simulink model "generic_20231123_1032"  (R2022b)
settings: Solver=ode45  StartTime=0.0  StopTime=50  RelTol=1e-3  EnableMultiTasking=on
model workspace (MAT data in the model file):
  A = 1
  Amplifier = -9.10007585438
  B = 1.19071237887
  K_d_yawrate = 0.231634180251
  K_dsteering = 5.24463953925
  k_speed = -0.570636497542
  k_stanley = 28.4909595466
  kd = -9.99955278144
  ki = 0.00519416981022
  kp = 9.99999979837
  path_curvature = 0
values from neighbouring files (symbols this model uses):
  brake_select = ones(length(speed), length(steering_angle))    [TwoDLook_uptable.m]
  curvature = 0.000:0.001:1    [TwoDLook_uptable.m]
  m = 1600    [MPCController1.m]    (also in MPCController2.m; MPC_Fmincon.m)
  speed = 0:0.1:100    [TwoDLook_uptable.m]
  steering_angle = -3.14/4:0.00628/4:3.14/4    [TwoDLook_uptable.m]
undefined symbols (not defined in the file or in its folder): DiscIntNeverNeededParam
libraries: CarMaker4SL x143, simulink x11, cstblocks x6, simulink_extras x4, autolibshared x1, mpcadaslib x1
(part 5 of 7)

== system generic_20231123_1032/CarMaker/VehicleControl/CreateBus VhclCtrl/Stanley steering & speed//Brake controller/Road sensor set & path planning/Road sensor set & path planning/Dijkestra path planning/Signal_smoothing/Smoothing4 ==
  Signal_In : Inport
  Add : Sum  Inputs=++++
  Delay : Delay  InitialCondition=0.1
  Delay1 : Delay  DelayLength=4  InitialCondition=0.1
  Delay2 : Delay  DelayLength=5  InitialCondition=0.1
  Gain : Gain  Gain=0.35
  Gain1 : Gain  Gain=0.25
  Gain2 : Gain  Gain=0.25
  Gain3 : Gain  Gain=0.15
  Signal_Out : Outport  VectorParamsAs1DForOutWhenUnconnected=off
  wires:
  Gain3/1 -> Add/4
  Delay2/1 -> Gain3/1
  Gain2/1 -> Add/3
  Add/1 -> Signal_Out/1, Delay/1, Delay1/1, Delay2/1
  Delay1/1 -> Gain2/1
  Gain/1 -> Add/1
  Delay/1 -> Gain1/1
  Signal_In/1 -> Gain/1
  Gain1/1 -> Add/2

== system generic_20231123_1032/CarMaker/VehicleControl/CreateBus VhclCtrl/Stanley steering & speed//Brake controller/Road sensor set & path planning/Road sensor set & path planning/Spline_path_planning/Signal_smoothing/Smoothing1 ==
  Signal_In : Inport
  Add : Sum  Inputs=++++
  Delay : Delay  InitialCondition=0.1
  Delay1 : Delay  DelayLength=4  InitialCondition=0.1
  Delay2 : Delay  DelayLength=5  InitialCondition=0.1
  Gain : Gain  Gain=0.35
  Gain1 : Gain  Gain=0.25
  Gain2 : Gain  Gain=0.25
  Gain3 : Gain  Gain=0.15
  Signal_Out : Outport  VectorParamsAs1DForOutWhenUnconnected=off
  wires:
  Gain1/1 -> Add/2
  Signal_In/1 -> Gain/1
  Delay/1 -> Gain1/1
  Gain/1 -> Add/1
  Delay1/1 -> Gain2/1
  Add/1 -> Delay2/1, Delay1/1, Delay/1, Signal_Out/1
  Gain2/1 -> Add/3
  Delay2/1 -> Gain3/1
  Gain3/1 -> Add/4

== system generic_20231123_1032/CarMaker/VehicleControl/CreateBus VhclCtrl/Stanley steering & speed//Brake controller/Road sensor set & path planning/Road sensor set & path planning/Spline_path_planning/Signal_smoothing/Smoothing2 ==
  Signal_In : Inport
  Add : Sum  Inputs=++++
  Delay : Delay  InitialCondition=0.1
  Delay1 : Delay  DelayLength=4  InitialCondition=0.1
  Delay2 : Delay  DelayLength=5  InitialCondition=0.1
  Gain : Gain  Gain=0.35
  Gain1 : Gain  Gain=0.25
  Gain2 : Gain  Gain=0.25
  Gain3 : Gain  Gain=0.15
  Signal_Out : Outport  VectorParamsAs1DForOutWhenUnconnected=off
  wires:
  Gain3/1 -> Add/4
  Delay2/1 -> Gain3/1
  Gain2/1 -> Add/3
  Add/1 -> Signal_Out/1, Delay/1, Delay1/1, Delay2/1
  Delay1/1 -> Gain2/1
  Gain/1 -> Add/1
  Delay/1 -> Gain1/1
  Signal_In/1 -> Gain/1
  Gain1/1 -> Add/2

== system generic_20231123_1032/CarMaker/VehicleControl/CreateBus VhclCtrl/Stanley steering & speed//Brake controller/Road sensor set & path planning/Road sensor set & path planning/Spline_path_planning/Signal_smoothing/Smoothing4 ==
  Signal_In : Inport
  Add : Sum  Inputs=++++
  Delay : Delay  InitialCondition=0.1
  Delay1 : Delay  DelayLength=4  InitialCondition=0.1
  Delay2 : Delay  DelayLength=5  InitialCondition=0.1
  Gain : Gain  Gain=0.35
  Gain1 : Gain  Gain=0.25
  Gain2 : Gain  Gain=0.25
  Gain3 : Gain  Gain=0.15
  Signal_Out : Outport  VectorParamsAs1DForOutWhenUnconnected=off
  wires:
  Gain1/1 -> Add/2
  Signal_In/1 -> Gain/1
  Delay/1 -> Gain1/1
  Gain/1 -> Add/1
  Delay1/1 -> Gain2/1
  Add/1 -> Delay2/1, Delay1/1, Delay/1, Signal_Out/1
  Gain2/1 -> Add/3
  Delay2/1 -> Gain3/1
  Gain3/1 -> Add/4

== system generic_20231123_1032/CarMaker/VehicleControl/CreateBus VhclCtrl/Stanley steering & speed//Brake controller/Road sensor set & path planning/Road sensor set & path planning/path_planning/Signal_smoothing/Smoothing1 ==
  Signal_In : Inport
  Add : Sum  Inputs=++++
  Delay : Delay  InitialCondition=0.1
  Delay1 : Delay  DelayLength=4  InitialCondition=0.1
  Delay2 : Delay  DelayLength=5  InitialCondition=0.1
  Gain : Gain  Gain=0.35
  Gain1 : Gain  Gain=0.25
  Gain2 : Gain  Gain=0.25
  Gain3 : Gain  Gain=0.15
  Signal_Out : Outport  VectorParamsAs1DForOutWhenUnconnected=off
  wires:
  Gain3/1 -> Add/4
  Delay2/1 -> Gain3/1
  Gain2/1 -> Add/3
  Add/1 -> Signal_Out/1, Delay/1, Delay1/1, Delay2/1
  Delay1/1 -> Gain2/1
  Gain/1 -> Add/1
  Delay/1 -> Gain1/1
  Signal_In/1 -> Gain/1
  Gain1/1 -> Add/2

== system generic_20231123_1032/CarMaker/VehicleControl/CreateBus VhclCtrl/Stanley steering & speed//Brake controller/Road sensor set & path planning/Road sensor set & path planning/path_planning/Signal_smoothing/Smoothing2 ==
  Signal_In : Inport
  Add : Sum  Inputs=++++
  Delay : Delay  InitialCondition=0.1
  Delay1 : Delay  DelayLength=4  InitialCondition=0.1
  Delay2 : Delay  DelayLength=5  InitialCondition=0.1
  Gain : Gain  Gain=0.35
  Gain1 : Gain  Gain=0.25
  Gain2 : Gain  Gain=0.25
  Gain3 : Gain  Gain=0.15
  Signal_Out : Outport  VectorParamsAs1DForOutWhenUnconnected=off
  wires:
  Gain1/1 -> Add/2
  Signal_In/1 -> Gain/1
  Delay/1 -> Gain1/1
  Gain/1 -> Add/1
  Delay1/1 -> Gain2/1
  Add/1 -> Delay2/1, Delay1/1, Delay/1, Signal_Out/1
  Gain2/1 -> Add/3
  Delay2/1 -> Gain3/1
  Gain3/1 -> Add/4

== system generic_20231123_1032/CarMaker/VehicleControl/CreateBus VhclCtrl/Stanley steering & speed//Brake controller/Road sensor set & path planning/Road sensor set & path planning/path_planning/Signal_smoothing/Smoothing4 ==
  Signal_In : Inport
  Add : Sum  Inputs=++++
  Delay : Delay  InitialCondition=0.1
  Delay1 : Delay  DelayLength=4  InitialCondition=0.1
  Delay2 : Delay  DelayLength=5  InitialCondition=0.1
  Gain : Gain  Gain=0.35
  Gain1 : Gain  Gain=0.25
  Gain2 : Gain  Gain=0.25
  Gain3 : Gain  Gain=0.15
  Signal_Out : Outport  VectorParamsAs1DForOutWhenUnconnected=off
  wires:
  Gain3/1 -> Add/4
  Delay2/1 -> Gain3/1
  Gain2/1 -> Add/3
  Add/1 -> Signal_Out/1, Delay/1, Delay1/1, Delay2/1
  Delay1/1 -> Gain2/1
  Gain/1 -> Add/1
  Delay/1 -> Gain1/1
  Signal_In/1 -> Gain/1
  Gain1/1 -> Add/2

== system generic_20231123_1032/CarMaker/VehicleControl/CreateBus VhclCtrl/Stanley steering & speed//Brake controller/Stanley_controller_vfin/Stanley_controller_vfin/Stanley_standfort controller/Steady_state_yaw/Steady_state_yaw ==
  V : Inport
  Curvature : Inport  Port=2
  Constant : Constant  Value=1600.004
  Constant1 : Constant  Value=70551.0
  Constant3 : Constant  Value=1.488
  Constant4 : Constant  Value=1.487
  Constant5 : Constant
  Divide : Product  Inputs=*/
  Divide1 : Product  Inputs=*/
  Gain : Gain  Gain=180/pi()
  Product : Product  Inputs=3
  Product1 : Product
  Square : Math  Operator=square
  Sum : Sum  Inputs=|++
  Steady_state_yaw : Outport
  wires:
  Square/1 -> Product/1
  Constant4/1 -> Divide/1
  Constant5/1 -> Sum/1
  Constant3/1 -> Divide/2
  V/1 -> Square/1
  Divide/1 -> Sum/2
  Sum/1 -> Product1/2
  Constant/1 -> Product/2
  Curvature/1 -> Product/3
  Constant1/1 -> Gain/1
  Product/1 -> Divide1/1
  Product1/1 -> Divide1/2
  Divide1/1 -> Steady_state_yaw/1
  Gain/1 -> Product1/1

== matlab function generic_20231123_1032/CarMaker/VehicleControl/Subsystem/MATLAB Function ==
  data: currentPosition input; currentHeading output; nextWaypoint input; desiredHeading output; headingError output
function [currentHeading, desiredHeading, headingError] = calculateHeadingError(currentPosition, nextWaypoint)
    % Calculate current heading, desired heading, and heading error for Stanley controller
    % Inputs:
    %   - currentPosition: Current position of the vehicle [x, y] (single points)
    %   - nextWaypoint: Next waypoint on the path [x, y]
    % Outputs:
    %   - currentHeading: Current heading of the vehicle (in radians)
    %   - desiredHeading: Desired heading or reference angle (in radians)
    %   - headingError: Heading error (in radians)
    function angle = wrapToPi(angle)
    % Wrap angle to the range [-pi, pi]
    angle = mod(angle + pi, 2 * pi) - pi;
    end
    % Extract x and y coordinates from the current position
    x = currentPosition(1);
    y = currentPosition(2);
    
    % Calculate the vector from the vehicle to the next waypoint
    headingVector = nextWaypoint - [x, y];

    % Calculate the current heading
    currentHeading = atan2(headingVector(2), headingVector(1));
    disp(currentHeading)
    disp('next')
    % Calculate the desired heading (heading of the vector between the current position and next waypoint)
    desiredHeading = atan2(nextWaypoint(2) - y, nextWaypoint(1) - x);
    disp(desiredHeading)
    % Calculate heading error
    headingError = wrapToPi(desiredHeading - currentHeading);
end

== matlab function generic_20231123_1032/CarMaker/VehicleControl/CreateBus VhclCtrl/Stanley steering & speed//Brake controller/Stanley controller with path_planning/Stanley controller with path_planning/MATLAB Function ==
  data: path input; dev input; e output; yaw input; speed_act input; err_fr_axle output; cross_track_steering output; heading_err output; steering output
function [e, err_fr_axle, cross_track_steering, heading_err, steering]  = conversion(path,dev,yaw,speed_act)
%path = [path_x;path_y];
function distance = calc_distance(pt,v1,v2)
    vect = v1 - v2;
    p_to_vect = pt - v2;
    crossVP = cross(vect,p_to_vect);
    distance = norm(crossVP) / norm(vect) * crossVP(3)/abs(crossVP(3));
end

e = zeros(1);
cross_track_steering = zeros(1);
heading_err = zeros(1);
steering=zeros(1);
err_fr_axle = zeros(1);

k_exp = 1.3059;
k = 15.028 + speed_act^k_exp;
k_ref = 2.62;

% path_index = fix(k_path * speed_act);
% if path_index > 13
%     path_index = 13;
% end
% 
% P_prev = path(:,6 + path_index);
% P_next = path(:,7 + path_index);

fr_axle = [-1.488 0 0];
distances = sqrt((path(1,:) - 1.488).^2 + (path(2,:) - 0).^2);
% Find the index of the closest point on the path
[~,err_fr_axle_ind] = min(distances);
if err_fr_axle_ind == 1
    err_fr_axle_ind = 2;
end
err_fr_axle = calc_distance(fr_axle,[path(1,err_fr_axle_ind - 1) path(2,err_fr_axle_ind - 1) 0],[path(1,err_fr_axle_ind) path(2,err_fr_axle_ind) 0]);

B = [-1.488 + k_ref * (speed_act / 27) 0 0];
distances_err = sqrt((path(1,:) - B(1)).^2 + (path(2,:) - 0).^2);
[~,err_ind] = min(distances_err);
if err_ind < 2
    err_ind = 2;
end
error = calc_distance(B,[path(1,err_ind - 1) path(2,err_ind - 1) 0],[path(1,err_ind) path(2,err_ind) 0]);


P_prev = path(:, err_ind-1);
P_next = path(:, err_ind);

x1 = P_prev(1,1);
y1 = P_prev(2,1);
x2 = P_next(1,1);
y2 = P_next(2,1);

a = (y2 - y1)/-(x2 + x1);
b = 1;
%c = -x1 * (y2 - y1) + y1 * (x2 - x1);


if speed_act ~= 0
    %e = c+b*y1/sqrt((a^2)+(b^2));
    e = error;
    
    cross_track_steering = atan(k * e / speed_act);
    heading_err = atan(-a / b) - yaw;
    %heading_err = 1/(tan(-a/b))-yaw;
    steering = heading_err + cross_track_steering;
end
end

== matlab function generic_20231123_1032/CarMaker/VehicleControl/CreateBus VhclCtrl/MPC_steering_controllers/Subsystem/MATLAB Function1 ==
  data: dev input; steering output; B input
function steering = advanced_speed_control_mpc(dev,B)
    % Model Predictive Controller (MPC) for speed contol
    % Define MPC parameters
    Ts = 0.1;  % Sampling time
    N = 10;    % Prediction horizon
    Q = 1;     % State weight
    R = 1;     % Input weight
    S = 0.1;   % Terminal state weight (integral term)
    
    % State-space model (simplified for illustration)
    %A = 0.8;
    %B = Ts;
    
    % Define cost and constraints for fmincon
    costFunction = @(u) (dev + B * u)' * Q * (dev + B * u) + u' * R * u + S * sum(u);
    Aeq = [];
    Beq = [];
    Aineq = [];
    Bineq = [];
    lb = -3.14; % Lower bound on throttle
    ub = 3.14;  % Upper bound on throttle
    
    % Steady-state error constraint
    Aineq = [Aineq; B];
    Bineq = [Bineq; -dev];
    
    % Initial guess
    u0 = 0;
    
    % Solve optimization problem
    options = optimoptions('fmincon', 'Display', 'off', 'Algorithm', 'sqp');
    u_opt = fmincon(costFunction, u0, Aineq, Bineq, Aeq, Beq, lb, ub, [], options);
    
    % Extract control input (throttle) from the optimization result
    steering = u_opt;
end

== matlab function generic_20231123_1032/CarMaker/VehicleControl/CreateBus VhclCtrl/Stanley steering & speed//Brake controller/Stanley_controller_with_thottle_and_brake_commands/Stanley steering + PID speed controller/Speed_controller/calculate_path_curvature ==
  data: path input; path_curvature output size=[1 20]; min_safe_speed output size=[1 20]; velocity_y input; velocity_x input; steering_angel input
function [path_curvature, min_safe_speed] = calculate_path_curvature(path,velocity_y,velocity_x,steering_angel)
    v_x = velocity_x* ones(1,20);
    v_y = velocity_y*ones(1,20);
    x = path(1,:)+v_x;
    y = path(2,:)+v_y;
    % First and second derivatives
    dx = gradient(x);
    dy = gradient(y);
    
    ddx = gradient(dx);
    ddy = gradient(dy);
    
    % Path curvature
    path_curvature = (dx .* ddy - dy .* ddx) ./ (dx.^2 + dy.^2).^(3/2);
    R = sqrt(1.61^2 +(1.61+1.28)^2*cot(steering_angel)^2)/12;
    % Minimum safe speed
    g = 9.81; % gravitational acceleration
    if max(path_curvature)>0.001 || max(path_curvature)<-0.001

        min_safe_speed = sqrt(g ./ abs(path_curvature));
    else
        min_safe_speed = sqrt(g .* abs(path_curvature));
end

== matlab function generic_20231123_1032/CarMaker/VehicleControl/CreateBus VhclCtrl/Stanley steering & speed//Brake controller/Stanley_controller_with_thottle_and_brake_commands/Stanley steering + PID speed controller/Stanely_controller ==
  data: dev_angle input; dev input; x1 input; x2 input; y1 input; y2 input; speed_act input; e output; cross_track_steering output; steering output
function [e, cross_track_steering, steering]  = conversion(dev_angle,dev, x1,x2,y1,y2,speed_act)


e = zeros(1);
cross_track_steering = zeros(1);


k_exp = 1.36;
k_def = 6;
k = k_def + abs(speed_act)^k_exp;

% Perform linear regression to find a, b, and c
% X = [path(1, :); path(2, :); ones(1, 20)]';  % Create a matrix for linear regression
% coefficients = X \ -1 * ones(20, 1);
% 
% % Extract the coefficients a, b, and c
% a = coefficients(1);
% b = coefficients(2);
% c = coefficients(3);
if (x2 ==0 && x1 ==0)|| x2==x1
a = 0;
b = 1;
c = y2+a*x2;
else
a = -(y2 - y1)/(x2-x1);
b = 1;
c = y2+a*x2;
end

if speed_act ~=0
    %e =abs(a*x_car+b*y_car+c)\sqrt(a^2+b^2); %abs(Dev_dis);
    e =-1*dev;% deviation distance
    cross_track_steering = atan(e*k / (1+speed_act));
    %heading_err = atan(-a/b)-yaw;
    heading_err = dev_angle; % heading error OR deviation angle
    steering = heading_err + cross_track_steering;

else
    steering = 0;
end
end

== matlab function generic_20231123_1032/CarMaker/VehicleControl/CreateBus VhclCtrl/MPC_steering_controllers/Subsystem/MATLAB Function5 ==
  data: x input; u input; u_optimal output; dt input; delta output; v_longitudinal output; path_ref input
function [u_optimal, delta, v_longitudinal] = MPCControllerPathTrackingWithHeadingError(x, u, dt,path_ref)
    function lateral_deviation = calculateLateralDeviation(x, path_ref)
        % Calculate lateral deviation from the reference path
        x_ref = path_ref(1, :);
        y_ref = path_ref(2, :);
    
        x_car = x(3);  % Lateral position of the car
        y_car = x(4);  % Yaw angle of the car
    
        % Rotate the car's coordinates to the reference path frame
        x_car_rot = cos(-x(4)) * (x_car - x_ref) - sin(-x(4)) * (y_car - y_ref);
        y_car_rot = sin(-x(4)) * (x_car - x_ref) + cos(-x(4)) * (y_car - y_ref);
    
        % Calculate lateral deviation
        lateral_deviation = y_car_rot;
    end
    % Adaptive Model Predictive Controller (Adaptive MPC) for steering control
    % Define system parameters (replace these with your actual vehicle parameters)
    lf = 1.449;  % Distance from centre of gravity to the front axle [m]
    m = 1600.0; % Kg
    lr = 1.449;   % Distance from centre of gravity to the Rear axle  [m]
    I = m*(lf+lr)^2/12;   % Carbody.inertia.z [Kgm2], assuming a rectangular shape
    theta = [0.1; 0.1];
    alpha = 0.1;
    cr = 160000; % Slip stiffness rear axle [N/rad]
    cf = 100000; % Slip stiffness Front axle [N/rad]
    % Define MPC parameters (modify as needed)
    N = 5;  % Prediction horizon
    Q = diag([1, 1, 10, 1, 1]);  % State cost matrix (including heading error)
    R = diag([0.1, 0.1]);  % Input cost matrix

    % Define state-space model
    A = [-2 * (cf + cr) / (m * u(2)), -u(2) - 2 * (cf * lf - cr * lr) / (m * u(2)); ...
         -2 * (cf * lf - cr * lr) / (m * u(2)), -2 * (cf * lf^2 + cr * lr^2) / (m * u(2))];
    B = [2 * cf / m, 0; 2 * cf * lf / (m * u(2)), 0];

    % Construct matrices for quadratic programming
    Qbar = blkdiag(kron(eye(N), Q), eye(N));  % State cost matrix for prediction horizon
    Rbar = kron(eye(N), R);  % Input cost matrix for prediction horizon
    
    % Ensure Qbar has the correct size
    Qbar = reshape(Qbar, [size(Qbar, 1), size(Qbar, 2)]);
    
    % Ensure x has the correct size
    x = reshape(x, [numel(x), 1]);
    
    % Initialize the Hessian matrix
    H = zeros(size(B, 2), size(B, 2));
    disp(Q)
    % Perform element-wise multiplication for each block in Qbar
    for i = 1:N
        H = H + B' * Qbar((i-1)*size(Q, 1) + 1:i*size(Q, 1), (i-1)*size(Q, 2) + 1:i*size(Q, 2)) * B;
    end

    % Add the Rbar term
    H = H + Rbar(1:2, 1:2);
    
    % Ensure x has the correct size for element-wise multiplication
    x = reshape(x, [numel(x), 1]);
    
    % Initialize the linear term
    f = zeros(size(B, 2), 1);
    
    % Perform element-wise multiplication for each block in Qbar
    for i = 1:N
        f = f + B' * Qbar((i-1)*size(Q, 1) + 1:i*size(Q, 1), (i-1)*size(Q, 2) + 1:i*size(Q, 2)) * x;
    end
    
    % Ensure f has the correct size
    f = reshape(f, [numel(f), 1]);


    % Define inequality constraints for longitudinal velocity
    Aineq = [0, 1; 0, -1];
    Bineq = [5 - u(2); u(2) - 5];

    % Solve quadratic programming problem
    options = optimoptions('fmincon', 'Display', 'off', 'Algorithm', 'sqp');
    % Initialize delta_u
    u0 = zeros(size(B, 2), 1);
    
    % Solve quadratic programming problem using fmincon
    delta_u = fmincon(@(u) 0.5 * u' * H * u + f' * u, u0, Aineq, Bineq, [], [], [], [], [], options);
    
    % Extract the optimal input from the solution
    u_optimal = delta_u(1:2);



    % Initialize x_new
    x_new = x;
    
    % Update state using the model
    x_new(1:2) = x_new(1:2) + (A(1:2, 1:2) * x(1:2) + B(1:2, :) * u_optimal) * dt;
    x_new(3:4) = x_new(3:4) + (A(3:4, 3:4) * x_new(3:4) + B(3:4, :) * u_optimal) * dt;
    
    % Initialize x_next
    x_next = zeros(size(x_new));
    
    % Adaptive parameter update (gradient descent)
    x_next(1:2) = x_new(1:2) + (A(1:2, 1:2) * x_new(1:2) + B(1:2, :) * u_optimal) * dt;
    x_next(3:4) = x_next(3:4) + (A(3:4, 3:4) * x_next(3:4) + B(3:4, :) * u_optimal) * dt;
    
    theta_new = theta - alpha * ((x_next(1:2) - x_new(1:2)) * x(1:2)');



    % Calculate lateral deviation from the reference path
    lateral_deviation = calculateLateralDeviation(x_new, path_ref);

    % Calculate heading error
    heading_error = x_new(4) - atan2(path_ref(2, end) - path_ref(2, 1), path_ref(1, end) - path_ref(1, 1));

    % Cost function modification for path tracking with heading error
    cost = lateral_deviation' * Q(3,3) * lateral_deviation + heading_error^2 + delta_u' * R * delta_u;

    % Extract control input (steering angle and longitudinal velocity) from the optimization result
    delta = u_optimal(1);
    v_longitudinal = u_optimal(2);

end

== matlab function generic_20231123_1032/CarMaker/VehicleControl/CreateBus VhclCtrl/Stanley steering & speed//Brake controller/Stanley_controller_with_thottle_and_brake_commands/Stanley steering + PID speed controller/Subsystem1/MATLAB Function ==
  data: u input; curv output; min_safe_speed input; speed output
function [curv, speed] = fcn(u, min_safe_speed)

curv = abs(max(u));
speed = max(min_safe_speed);

== matlab function generic_20231123_1032/CarMaker/VehicleControl/CreateBus VhclCtrl/MPC_steering_controllers/Subsystem/MATLAB Function3 ==
  data: x input; u input; u_optimal output; dt input; x_new output; theta_new output
function [u_optimal, x_new,theta_new] = adaptive_steering_mpc(x,u,dt)
    % Adaptive Model Predictive Controller (Adaptive MPC) for steering control
    % Define system parameters (replace these with your actual vehicle parameters)
    lf = 1.449;  % Distance from centre of gravity to the front axle [m]
    lr = 1.449;   % Distance from centre of gravity to the Rear axle  [m]
    I = m*(lf+lr)^2/12;   % Carbody.inertia.z [Kgm2], assuming a rectangular shape
    
    cr = 160000; % Slip stiffness rear axle [N/rad]
    cf = 100000; % Slip stiffness Front axle [N/rad]
    % Define MPC parameters (modify as needed)
    N = 5;  % Prediction horizon
    Q = eye(4);  % State cost matrix
    R = eye(2);  % Input cost matrix

    % Define state-space model
    A = [-2 * (cf + cr) / (m * u(2)), -u(2) - 2 * (cf * lf - cr * lr) / (m * u(2)); ...
         -2 * (cf * lf - cr * lr) / (m * u(2)), -2 * (cf * lf^2 + cr * lr^2) / (m * u(2))];
    B = [2 * cf / m, 0; 2 * cf * lf / (m * u(2)), 0];

    % Construct matrices for quadratic programming
    Qbar = blkdiag(kron(eye(N), Q), eye(N));  % State cost matrix for prediction horizon
    Rbar = kron(eye(N), R);  % Input cost matrix for prediction horizon
    H = B' * Qbar * B + Rbar;  % Hessian matrix
    f = (x' * Qbar * B)';  % Linear term

    % Solve quadratic programming problem
    options = optimset('Display', 'off');
    delta_u = quadprog(H, f, [], [], [], [], [], [], [], options);

    % Extract the optimal input from the solution
    u_optimal = delta_u(1:2);

    % Update state using the model
    x_new = x + (A * x + B * u_optimal) * dt;

    % Adaptive parameter update (gradient descent)
    x_next = x_new + (A * x_new + B * u_optimal) * dt;
    theta_new = theta - alpha * (x_next - x_new) * x';
end

== matlab function generic_20231123_1032/CarMaker/VehicleControl/CreateBus VhclCtrl/MPC_steering_controllers/Subsystem/MATLAB Function4 ==
  data: heading_error input; delta output; u2 input
function delta = ampc_steering_control(heading_error, u2)
    persistent model_params
    function params = initialize_model_params()
        % Define the vehicle parameters
        m = 2100;  % Car body mass [Kg]
        lf = 1.2;  % Distance from center of gravity to the front axle [m]
        lr = 1.6;  % Distance from center of gravity to the rear axle [m]
        I = m * (lf + lr)^2 / 12;  % Car body inertia [Kgm^2]
    
        cr = 160000;  % Slip stiffness rear axle [N/rad]
        cf = 100000;  % Slip stiffness front axle [N/rad]
    
        % Define the state-space model
        A = [-2 * (cf + cr) / m, -u2; -2 * (cf * lf - cr * lr) / I, -2 * (cf * lf^2 + cr * lr^2) / I];
        B = [2 * cf / m; 2 * cf * lf / I];
    
        % Store parameters in a struct
        params.A = A;
        params.B = B;
    
        % Initialize adaptive parameters if needed
        % params.adaptive_param = ...
    
    end

    function updated_params = update_model_params(params, u2)
        % Implement adaptive parameter update if needed
        % Example:
        % params.adaptive_param = params.adaptive_param + 0.1 * (desired_value - measured_value);
        % ...
    
        % Return the updated parameters
        updated_params = params;
    end
    % Parameters
    Ts = 0.1;  % Sampling time
    N = 10;    % Prediction horizon

    % Update the model parameters if not initialized
    if isempty(model_params)
        model_params = initialize_model_params();
    end

    % State vector (simplified, assuming heading_error is the heading error)
    x = [heading_error; 0];

    % Define cost and constraints for fmincon
    costFunction = @(u) (x + model_params.A * x + model_params.B * u)' * (x + model_params.A * x + model_params.B * u);
    Aeq = [];
    Beq = [];
    Aineq = [];
    Bineq = [];
    lb = -1.5;  % Lower bound on steering input
    ub = 1.5;   % Upper bound on steering input

    % Initial guess
    u0 = 0;

    % Solve optimization problem to get optimal steering input
    options = optimoptions('fmincon', 'Display', 'off', 'Algorithm', 'sqp');
    u_opt = fmincon(costFunction, u0, Aineq, Bineq, Aeq, Beq, lb, ub, [], options);

    % Extract control input (steering angle) from the optimization result
    delta = u_opt;

    % Update model parameters adaptively
    model_params = update_model_params(model_params, u2);
end

== matlab function generic_20231123_1032/CarMaker/VehicleControl/CreateBus VhclCtrl/Stanley steering & speed//Brake controller/Stanley controller with path_planning/Stanley controller with path_planning/Path_Calculation_V02 ==
  data: x_car input; closest_point output; y_car input; path_x input; instantaneous_path output; y_path input
function [closest_point, instantaneous_path] = calculate_path(x_car, y_car, path_x, y_path)
% x_car: x position of the car
% y_car: y position of the car
% path: [2x400] matrix representing the path
path = [path_x;y_path];
%Smoothing the Path
x = path(1,:);
y = path(2,:);
% Define the number of points you want to add for interpolation
num_extra_points = 10000; % Adjust this value as per your requirements
% Compute the total number of points after interpolation
total_points = numel(x) + num_extra_points;
existing_indices = 1:numel(x);
% Create an array of indices for the interpolated points
interpolated_indices = linspace(1, numel(x), total_points);
% Perform spline interpolation on both x and y coordinates
x_interpolated = spline(existing_indices, x, interpolated_indices);
y_interpolated = spline(existing_indices, y, interpolated_indices);

smoothed_path =vertcat(x_interpolated, y_interpolated);
% smoothed_path = smoothed_path_t';


% Calculate the distance between the car and each point on the path
distances = sqrt((smoothed_path(1,:) - x_car).^2 + (smoothed_path(2,:) - y_car).^2);

% Find the index of the closest point on the path
[~, closest_index] = min(distances);

% Get the closest point on the path
closest_point = smoothed_path(:, closest_index);

% Calculate the distance from the closest point to the beginning of the path
distance_to_start = sqrt(sum((smoothed_path(:,closest_index) - smoothed_path(:,1)).^2));

% Calculate the distance from the closest point to the end of the path
distance_to_end = sqrt(sum((smoothed_path(:,closest_index) - smoothed_path(:,end)).^2));

% Determine the number of points to include in the instantaneous path
num_points = min(size(smoothed_path, 2), 20);

% Initialize the instantaneous_path variable using coder.nullcopy
instantaneous_path = coder.nullcopy(zeros(2, num_points));

if distance_to_start < distance_to_end
    % If the closest point is closer to the beginning of the path than the
    % end, include the points starting from the closest point towards the
    % end of the path
    start_index = closest_index;
    end_index = min(size(smoothed_path, 2), closest_index+num_points-1);
else
    % If the closest point is closer to the end of the path than the
    % beginning, include the points starting from the closest point towards
    % the beginning of the path
    start_index = max(1, closest_index-num_points+1);
    end_index = closest_index;
end

%own 
start_index = closest_index;
if start_index > 11139
    end_index = 11159;
    if start_index > 11149
        start_index = 0;
        end_index=20;
    end
else
    end_index = min(size(smoothed_path, 2), closest_index+num_points-1);
end
%own

temp_path = smoothed_path(:, start_index:end_index);
instantaneous_path(:, num_points-size(temp_path, 2)+1:num_points) = temp_path;

end

== matlab function generic_20231123_1032/CarMaker/VehicleControl/CreateBus VhclCtrl/Stanley steering & speed//Brake controller/Stanley controller with path_planning/Stanley controller with path_planning/MATLAB Function1 ==
  data: Pos_X input; Path_Out output; Pos_Y input; Yaw_Angle input; Path_In input
function Path_Out = Abs2RelNew(Pos_X, Pos_Y, Yaw_Angle, Path_In)
%Rotation matrix from absolute to relativ coordination system
R = [cos(Yaw_Angle) sin(Yaw_Angle); -sin(Yaw_Angle) cos(Yaw_Angle)];

Path_X=Path_In(1,:)-Pos_X;      % Shift the points in to the car position
Path_Y=Path_In(2,:)-Pos_Y;      % Shift the points in to the car position
Path=[Path_X;Path_Y];           % Car Point
Path_Out = R*Path;              % Rotate the shifted Points

== matlab function generic_20231123_1032/CarMaker/VehicleControl/Estimate object diemnsions/MATLAB Function ==
  data: range input; estimatedWidth output; azimuth input; elevation input; sensorFOV input; estimatedHeight output; sensorHeight input
function [estimatedWidth, estimatedHeight] = estimateObjectDimensions(range, azimuth, elevation, sensorFOV, sensorHeight)
    % Estimate object dimensions based on perspective projection

    % Assuming sensorFOV is in degrees
    sensorFOV_horizontal = deg2rad(sensorFOV(1));
    sensorFOV_vertical = deg2rad(sensorFOV(2));

    % Adjusted width and height based on perspective projection
    adjustedWidth =  range * tan(sensorFOV_horizontal / 2);
    adjustedHeight =   range * tan(sensorFOV_vertical / 2);

    % Adjust dimensions based on azimuth and elevation
    % For simplicity, assuming azimuth and elevation are angles in radians
    % You may need to adjust based on your sensor's coordinate system

    % Width adjustment based on azimuth
    adjustedWidth = adjustedWidth * cos(azimuth*22.5);

    % Height adjustment based on elevation
    adjustedHeight = adjustedHeight * cos(elevation*22.5);

    % Correct for perspective distortion based on sensor height
   % if sensorHeight > 0
        %perspectiveFactor = sensorHeight / range;
        %adjustedWidth = adjustedWidth * perspectiveFactor;
        %adjustedHeight = adjustedHeight * perspectiveFactor;
  %end

    estimatedWidth = adjustedWidth;
    estimatedHeight = adjustedHeight;
end

== matlab function generic_20231123_1032/CarMaker/VehicleControl/Subsystem1/Obstacle_data_gathering/MATLAB Function6 ==
  data: path_dev input; error output; y_dev input; y_error3 input; y_error_2 input; y_error input; distance input; x_distance_obj input
function error= fcn(path_dev, y_dev, y_error3, y_error_2, y_error, distance, x_distance_obj)
if distance <15 && distance >1
    %if y_error >0 || y_error_2 >0 || y_error3 >0
    %error =-(path_dev+y_dev/2);
    %else
        error =path_dev-y_dev/2;
elseif distance <1 && distance >-4
    error =path_dev/4-y_dev/2;
elseif (distance <-5 && distance >-8) && x_distance_obj >0
    error = -path_dev/4;
elseif distance <-6 && distance >-11.5
    error = -path_dev + path_dev/1.69; % path_dev - something_ (positve->0 when the we are not near the object
else
    error = path_dev;
end
end

== matlab function generic_20231123_1032/CarMaker/VehicleControl/Subsystem1/Obstacle_data_gathering/MATLAB Function8 ==
  data: y_added output; y_dev input; data input; distance input
function y_added= fcn( y_dev, data, distance)
if distance <12 && distance >-4
   y_added = data+y_dev;
else
    y_added = 0;
end
end

== matlab function generic_20231123_1032/CarMaker/VehicleControl/CreateBus VhclCtrl/MATLAB Function1 ==
  data: e input; steering output; Cf input; Cr input; v input
function steering = fcn(e,Cf,Cr,v)
%lf = 1.488
%lr = 1.487;
%Cf = 
%Cr =
%m =
% v = 
steering = ((lf+lr)- (lf*Cf-lr*Cr)*m*vx^2)*e...
    /(d_pre*(d_pre+2*L));

== matlab function generic_20231123_1032/CarMaker/VehicleControl/CreateBus VhclCtrl/path_planner_MATLAB/MATLAB Function1 ==
  data: u input; path_x output; path_y output; path_yaw output
function [path_x,path_y,path_yaw] = fcn(u)
path_x = u(1,:);
path_y = u(2,:);
path_yaw = u(3,:);
end

== matlab function generic_20231123_1032/CarMaker/VehicleControl/CreateBus VhclCtrl/path_planner_MATLAB/MATLAB Function ==
  data: path input; e output; yaw input; speed_act input; err_fr_axle output; cross_track_steering output; heading_err output; steering output
function [e, err_fr_axle, cross_track_steering, heading_err, steering]  = conversion(path,yaw,speed_act)
%path = [path_x;path_y];
function distance = calc_distance(pt,v1,v2)
    vect = v1 - v2;
    p_to_vect = pt - v2;
    crossVP = cross(vect,p_to_vect);
    distance = norm(crossVP) / norm(vect) * crossVP(3)/abs(crossVP(3));
end

e = zeros(1);
cross_track_steering = zeros(1);
heading_err = zeros(1);
steering=zeros(1);
err_fr_axle = zeros(1);

k_exp = 1.36;
k_def = 6;
k = k_def + abs(speed_act)^k_exp;
k_ref = 3.1;

% path_index = fix(k_path * speed_act);
% if path_index > 13
%     path_index = 13;
% end
% 
% P_prev = path(:,6 + path_index);
% P_next = path(:,7 + path_index);

fr_axle = [-1.488 0 0];
distances = sqrt((path(1,:) - 1.488).^2 + (path(2,:) - 0).^2);
% Find the index of the closest point on the path
[~,err_fr_axle_ind] = min(distances);
if err_fr_axle_ind == 1
    err_fr_axle_ind = 2;
end
err_fr_axle = calc_distance(fr_axle,[path(1,err_fr_axle_ind - 1) path(2,err_fr_axle_ind - 1) 0],[path(1,err_fr_axle_ind) path(2,err_fr_axle_ind) 0]);

B = [-1.488 + k_ref * (speed_act / 27) 0 0];
distances_err = sqrt((path(1,:) - B(1)).^2 + (path(2,:) - 0).^2);
[~,err_ind] = min(distances_err);
if err_ind < 2
    err_ind = 2;
end
error = calc_distance(B,[path(1,err_ind - 1) path(2,err_ind - 1) 0],[path(1,err_ind) path(2,err_ind) 0]);


P_prev = path(:, err_ind-1);
P_next = path(:, err_ind);

x1 = P_prev(1,1);
y1 = P_prev(2,1);
x2 = P_next(1,1);
y2 = P_next(2,1);

a = (y2 - y1)/-(x2 + x1);
b = 1;
%c = -x1 * (y2 - y1) + y1 * (x2 - x1);


if speed_act ~= 0
    %e = c+b*y1/sqrt((a^2)+(b^2));
    e = error;
    
    cross_track_steering = atan(k * e / speed_act);
    heading_err = atan(-a / b) - yaw;
    %heading_err = 1/(tan(-a/b))-yaw;
    steering = heading_err + cross_track_steering;
end
end

== matlab function generic_20231123_1032/CarMaker/VehicleControl/CreateBus VhclCtrl/path_planner_MATLAB/MATLAB Function2 ==
  data: Pos_X input; Path_Out output; Pos_Y input; Yaw_Angle input; Path_In input
function Path_Out = Abs2RelNew(Pos_X, Pos_Y, Yaw_Angle, Path_In)
%Rotation matrix from absolute to relativ coordination system
R = [cos(Yaw_Angle) sin(Yaw_Angle); -sin(Yaw_Angle) cos(Yaw_Angle)];

Path_X=Path_In(1,:)-Pos_X;      % Shift the points in to the car position
Path_Y=Path_In(2,:)-Pos_Y;      % Shift the points in to the car position
Path=[Path_X;Path_Y];           % Car Point
Path_Out = R*Path;              % Rotate the shifted Points

== matlab function generic_20231123_1032/CarMaker/VehicleControl/CreateBus VhclCtrl/path_planner_MATLAB/Path_Calculation_V02 ==
  data: x_car input; closest_point output; y_car input; path_x input; instantaneous_path output; y_path input
function [closest_point, instantaneous_path] = calculate_path(x_car, y_car, path_x, y_path)
% x_car: x position of the car
% y_car: y position of the car
% path: [2x400] matrix representing the path
path = [path_x;y_path];
%Smoothing the Path
x = path(1,:);
y = path(2,:);
% Define the number of points you want to add for interpolation
num_extra_points = 0; % Adjust this value as per your requirements
% Compute the total number of points after interpolation
total_points = numel(x) + num_extra_points;
existing_indices = 1:numel(x);
% Create an array of indices for the interpolated points
interpolated_indices = linspace(1, numel(x), total_points);
% Perform spline interpolation on both x and y coordinates
x_interpolated = spline(existing_indices, x, interpolated_indices);
y_interpolated = spline(existing_indices, y, interpolated_indices);

smoothed_path =vertcat(x_interpolated, y_interpolated);
% smoothed_path = smoothed_path_t';


% Calculate the distance between the car and each point on the path
distances = sqrt((smoothed_path(1,:) - x_car).^2 + (smoothed_path(2,:) - y_car).^2);

% Find the index of the closest point on the path
[~, closest_index] = min(distances);

% Get the closest point on the path
closest_point = smoothed_path(:, closest_index);

% Calculate the distance from the closest point to the beginning of the path
distance_to_start = sqrt(sum((smoothed_path(:,closest_index) - smoothed_path(:,1)).^2));

% Calculate the distance from the closest point to the end of the path
distance_to_end = sqrt(sum((smoothed_path(:,closest_index) - smoothed_path(:,end)).^2));

% Determine the number of points to include in the instantaneous path
num_points = min(size(smoothed_path, 2), 20);

% Initialize the instantaneous_path variable using coder.nullcopy
instantaneous_path = coder.nullcopy(zeros(2, num_points));

if distance_to_start < distance_to_end
    % If the closest point is closer to the beginning of the path than the
    % end, include the points starting from the closest point towards the
    % end of the path
    start_index = closest_index;
    end_index = min(size(smoothed_path, 2), closest_index+num_points-1);
else
    % If the closest point is closer to the end of the path than the
    % beginning, include the points starting from the closest point towards
    % the beginning of the path
    start_index = max(1, closest_index-num_points+1);
    end_index = closest_index;
end

%own 
start_index = closest_index;
if start_index > 11139
    end_index = 11159;
    if start_index > 11149
        start_index = 0;
        end_index=20;
    end
else
    end_index = min(size(smoothed_path, 2), closest_index+num_points-1);
end
%own

temp_path = smoothed_path(:, start_index:end_index);
instantaneous_path(:, num_points-size(temp_path, 2)+1:num_points) = temp_path;

end

== matlab function generic_20231123_1032/CarMaker/VehicleControl/CreateBus VhclCtrl/A*algoithm/MATLAB Function1 ==
  data: start input; deviation output; target input; obstacles input; pathX output; pathY output
function [deviation, pathX, pathY] = generatePathWithObstacles(start, target, obstacles)
    % A* Path Planning
    function path = astar(start, goal, obstacles)
    % A* algorithm implementation
    
    function path = reconstructPath(parent, current)
    % Reconstruct the path from the parent array
    path_old = current;
    while any(parent(:, 1) == path_old(1) & parent(:, 2) == path_old(2))
        idx = find(parent(:, 1) == path_old(1) & parent(:, 2) == path_old(2), 1);
        path = [parent(idx, :); path_old];
    end
    path = path_old;
end
    function neighbors = generateNeighbors(current, obstacles)
    % Generate neighboring nodes (adjacent and diagonal)
    possibleMoves = [-1, 0; 1, 0; 0, -1; 0, 1; -1, -1; -1, 1; 1, -1; 1, 1];
    neighbors = bsxfun(@plus, current, possibleMoves);

    % Filter out neighbors outside the map
    inMap = neighbors(:, 1) >= 1 & neighbors(:, 1) <= 100 & neighbors(:, 2) >= 1 & neighbors(:, 2) <= 100;
    neighbors = neighbors(inMap, :);
    end
    function result = inSet(position, set)
    % Check if a position is in the set
    result = any(isequal(set(:, 1:2), position), 2);
end

    function result = inObstacles(position, obstacles)
    % Check if a position is in the obstacles
    result = any(isequal(obstacles, position), 2);
    end
    % Parameters
    mapSize = 100; % Adjust as needed
    openSet = zeros(mapSize, 3); % [x, y, f]
    closedSet = zeros(mapSize, 3); % [x, y, f]
    parent = zeros(mapSize, 2); % [parentX, parentY]

    % Functions to calculate heuristic and cost
    heuristic = @(pos, goal) sqrt((pos(1) - goal(1))^2 + (pos(2) - goal(2))^2);
    cost = @(pos, parent) sqrt((pos(1) - parent(1))^2 + (pos(2) - parent(2))^2);

    % Initialize starting point
    openSet(1, :) = [start, heuristic(start, goal)];
    closedSet = zeros(mapSize, 3);

    while any(openSet(:, 1))
        % Find the node with the lowest f in the open set
        [~, currentIdx] = min(openSet(:, 3));
        current = openSet(currentIdx, 1:2);

        % Goal reached
        if isequal(current, goal)
            path = reconstructPath(parent, current);
            return;
        end

        % Move current from openSet to closedSet
        openSet(currentIdx, :) = [0, 0, 0];
        closedSet(currentIdx, :) = [current, heuristic(current, goal)];

        % Generate neighbors
        neighbors = generateNeighbors(current, obstacles);

        for i = 1:size(neighbors, 1)
            neighbor = neighbors(i, :);

            % Skip if in closedSet or obstacle
            if ~inSet(neighbor, closedSet) && ~inObstacles(neighbor, obstacles)
                % Calculate tentative g score
                tentativeG = cost(neighbor, current) + cost(current, start);

                % Check if neighbor is not in openSet or has a better g score
                idxInOpenSet = find(isequal(openSet(:, 1:2), neighbor), 1);
                if isempty(idxInOpenSet) || tentativeG < cost(neighbor, start)
                    % Update parent and g score
                    parent(idxInOpenSet, :) = current;
                    openSet(idxInOpenSet, :) = [neighbor, tentativeG + heuristic(neighbor, goal)];
                end
            end
        end
    end

    % No path found
    path = [];
end
    path = astar(start, target, obstacles);

    % Extract X and Y coordinates from the path
    pathX1 = path(:, 1);
    pathX = pathX1(1);
    pathY1 = path(:, 2);
    pathY = pathY1(1);

    % Calculate deviation from the vehicle to the generated path
    deviation_1 = sqrt((start(1) - pathX).^2 + (start(2) - pathY).^2);
    deviation =deviation_1(1); 
end

== matlab function generic_20231123_1032/CarMaker/VehicleControl/Subsystem/MATLAB Function1 ==
  data: x input; path output; y input
function path = fcn(x , y)
path = [x;y];
end

== matlab function generic_20231123_1032/CarMaker/VehicleControl/Subsystem1/MATLAB Function ==
  data: vehicleX input; deviationAngle output; vehicleY input; pathX input; pathY input; vehicleYaw input
function deviationAngle = calculateDeviationAngle(vehicleX, vehicleY, pathX, pathY, vehicleYaw)
    % Calculate the vector from the vehicle to the path point
    vectorToPath = [pathX - vehicleX, pathY - vehicleY];

    % Calculate the angle between the vehicle's heading and the vector to the path point
    angleToPath = atan2(vectorToPath(2), vectorToPath(1));

    % Calculate the deviation angle
    deviationAngle = vehicleYaw - angleToPath;

    % Ensure the result is within the range [-pi, pi]
    deviationAngle = mod(deviationAngle + pi, 2*pi) - pi;
end

== matlab function generic_20231123_1032/CarMaker/VehicleControl/CreateBus VhclCtrl/Stanley steering & speed//Brake controller/Road sensor set & path planning/Road sensor set & path planning/Car_yaw_rate/calculate_path_curvature2 ==
  data: path_x input; path_curvature output; path_y input
function path_curvature = calculate_path_curvature(path_x, path_y)
    x = path_x;
    y = path_y;
    
    % First and second derivatives
    dx = gradient(x);
    dy = gradient(y);
    
    ddx = gradient(dx);
    ddy = gradient(dy);
    
    % Path curvature with a small constant added to the denominator
    epsilon = 1e-6; % small constant to avoid division by zero
    curvature_denominator = (dx.^2 + dy.^2).^(3/2) + epsilon;
    path_curvature = max((dx .* ddy - dy .* ddx) ./ curvature_denominator);
    
    % Smooth the curvature using a moving average
    window_size = 5; % adjust the window size as needed
    path_curvature = smoothdata(path_curvature, 'movmean', window_size);
end

== matlab function generic_20231123_1032/CarMaker/VehicleControl/CreateBus VhclCtrl.Steering/MATLAB Function1 ==
  data: dev_dest input; error output; y_car input; Y_dev input
function error = fcn(dev_dest, y_car, Y_dev)
if y_car <10 && y_car>0
    error = -y_car;

else
    error =dev_dest;
end
end

== matlab function generic_20231123_1032/CarMaker/VehicleControl/CreateBus VhclCtrl/Stanley steering & speed//Brake controller/Road sensor set & path planning/Road sensor set & path planning/Path_curvature/calculate_path_curvature1 ==
  data: path_x input; path_curvature output; path_y input
function path_curvature = calculate_path_curvature(path_x, path_y)
    x = path_x;
    y = path_y;
    
    % First and second derivatives
    dx = gradient(x);
    dy = gradient(y);
    
    ddx = gradient(dx);
    ddy = gradient(dy);
    
    % Path curvature with a small constant added to the denominator
    epsilon = 1e-6; % small constant to avoid division by zero
    curvature_denominator = (dx.^2 + dy.^2).^(3/2) + epsilon;
    path_curvature = max((dx .* ddy - dy .* ddx) ./ curvature_denominator);
    
    % Smooth the curvature using a moving average
    window_size = 5; % adjust the window size as needed
    path_curvature = smoothdata(path_curvature, 'movmean', window_size);
end

== matlab function generic_20231123_1032/CarMaker/VehicleControl/CreateBus VhclCtrl/Stanley steering & speed//Brake controller/Road sensor set & path planning/Road sensor set & path planning/Cross_track_error_calcuation/Cross_track_error_calcuation ==
  data: x_vehicle input; cte output; y_vehicle input; x_point input; y_point input; denominator output; x2 input; y2 input
function [cte,denominator]= calculate_cross_track_error(x_vehicle, y_vehicle, x_point, y_point,x2,y2)
    % Calculate cross-track error for a given vehicle position and single point
    function cte = calculate_perpendicular_distance(x_vehicle, y_vehicle, x_point, y_point)
    % Calculate the perpendicular distance from the vehicle to the point

    % Coordinates of the point
    x1 = x_point;
    y1 = y_point;
    %x2 = x_vehicle;
    %y2 = y_vehicle;

    % Calculate the cross-track error using the formula for the distance from a point to a line
    numerator = (x2 - x1) * (y1 - y_vehicle) - (x1 - x_vehicle) * (y2 - y1);
    denominator = sqrt((x2 - x1)^2 + (y2 - y1)^2);

    % Ensure that the denominator is not zero to avoid division by zero
    if denominator ~= 0
        cte = (numerator / denominator);
    else
        cte = 0;
    end
end
    % Calculate cross-track error as the perpendicular distance
    cte = calculate_perpendicular_distance(x_vehicle, y_vehicle, x_point, y_point);
end

== matlab function generic_20231123_1032/CarMaker/VehicleControl/CreateBus VhclCtrl/Stanley steering & speed//Brake controller/Road sensor set & path planning/Road sensor set & path planning/path_planning/Basic_obstacle avoidance ==
  data: Car_x input; updated_path output; Car_y input; dx input; dy input; object_width input; object_length input; path_x input; path_y input; car_v input; car_v_ceil input
function updated_path = obstacleAvoidanceSimulink(Car_x, Car_y, dx, dy, object_width, object_length, path_x, path_y,car_v, car_v_ceil)
    % Parameters
    if car_v >14
    safety_distance = car_v; % Adjust based on your requirements
    else
        safety_distance = 14;
    end
    %disp(car_v)
    % Check if the vehicle is close to the object
    distance_to_object = sqrt(dx^2 + dy^2);
    if (distance_to_object-object_length < safety_distance && distance_to_object > 0) && dx>0
        % Calculate the trajectory to avoid the entire obstacle
        angle_to_object = atan2(dy, dx);
        object_heading = atan2(object_length, object_width); % Assuming object is aligned with x-axis

        % Calculate new position to avoid the entire obstacle
        new_x = -1*(path_x + (car_v_ceil + object_length) * sin(angle_to_object + object_heading));
        new_y = -1*(path_y + (car_v_ceil + object_width/2) * cos(angle_to_object + object_heading));

        % Update the path to follow the new trajectory
        updated_path = [new_x; new_y] * ones(1, length(path_x));
    else
        updated_path = [path_x; path_y];
        %window_size = 5; % adjust the window size as needed
    %path_curvature = smoothdata(path_curvature, 'movmean', window_size)
    end
end
